simulink model "item3_simulink_motorCC_217947_222370"  (R2022a)
settings: Solver=VariableStepAuto  StartTime=0.0  StopTime=0.2  RelTol=1e-6
values from neighbouring files (symbols this model uses):
  Ia_placa = 25    [matlab_motorCC_217947_222370.m]
  J = 0.00252    [matlab_motorCC_217947_222370.m]
  K = Te_placa/Ia_placa    (= 0.424752712124)    [matlab_motorCC_217947_222370.m]
  Kac = 1/Kpc    (= 0.588235294118)    [matlab_motorCC_217947_222370.m]
  Kas = 1/Kps    (= 1.68552663541)    [matlab_motorCC_217947_222370.m]
  Kic = Ra*wcc    (= 260)    [matlab_motorCC_217947_222370.m]
  Kis = J*wcs^2/(5*K)    (= 11.8657276485)    [matlab_motorCC_217947_222370.m]
  Kpc = La*wcc    (= 1.7)    [matlab_motorCC_217947_222370.m]
  Kps = J*wcs/K    (= 0.593286382423)    [matlab_motorCC_217947_222370.m]
  La = 1.7e-3    (= 0.0017)    [matlab_motorCC_217947_222370.m]
  Ra = 0.26    [matlab_motorCC_217947_222370.m]
  Te_placa = Potencia/Wm_placa    (= 10.6188178031)    [matlab_motorCC_217947_222370.m]
  Va_placa = 140    [matlab_motorCC_217947_222370.m]
libraries: spsDCVoltageSourceLib x1, spsDCMachineLib x1, spsFullBridgeConverterLib x1, spsPWMGenerator2LevelLib x1, spspowerguiLib x1
settings Model: Creator=mathe  LastModifiedBy=Pichau

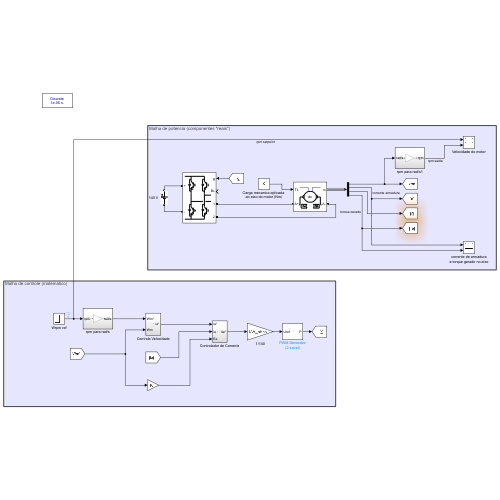
[thumbnail: Simulink's stored preview of the top-level diagram]
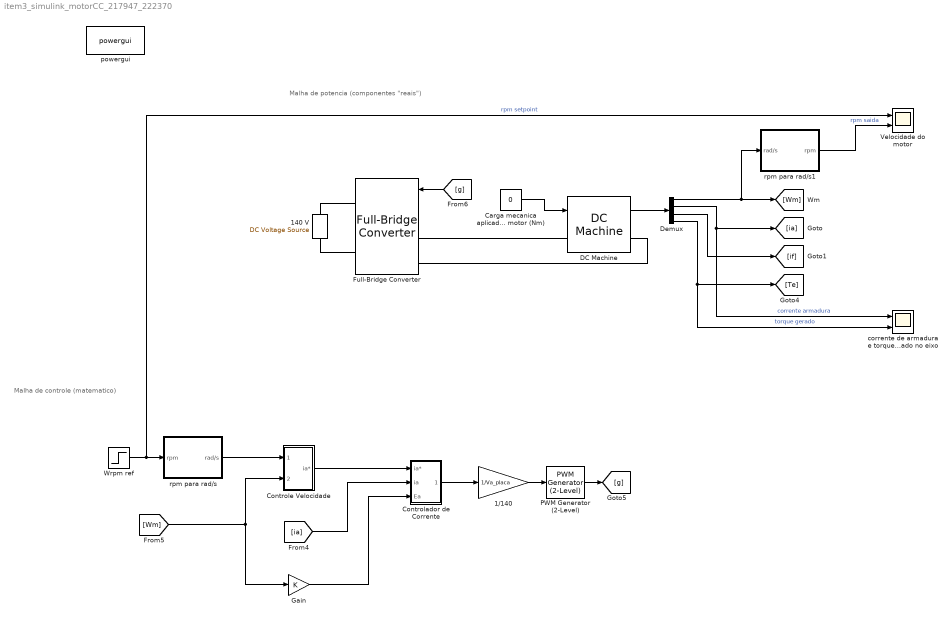
== system item3_simulink_motorCC_217947_222370 ==
  note: Malha de potencia (componentes "reais")
  note: Malha de controle (matematico)
  1/140 : Gain  Gain=1/Va_placa
  140 V : spsDCVoltageSourceLib/DC Voltage Source  Amplitude=Va_placa  Measurements=None
  Carga mecanica aplicada ao eixo do motor (Nm) : Constant  Value=0
  Controlador de Corrente : Subsystem
  Controle Velocidade : Subsystem
  DC Machine : spsDCMachineLib/DC Machine  PresetModel=No  MechanicalLoad=Torque TL  FieldType=Permanent magnet  ShowDetailedParameters=on  MeasurementBus=off  RLa="[ Ra  La]"  RLf="[ 240  120]"  Laf=1.8  MachineConstant=Torque constant (N.m/A)  Ke=1.8  Kt=K  J=J  Bm=B  Tf=0  w0=0  Ifinit=1  TsPowergui=0  TsBlock=-1
  Demux : Demux
  Full-Bridge Converter : spsFullBridgeConverterLib/Full-Bridge Converter  ModelType=Switching devices  Ron=1e-3  Rs=1e6  Cs=inf  Vforward=[0,0]  Ron_Diode=1e-3  Rs_Diode=1e6  Cs_Diode=inf  Vf_Diode=1e-3  Rs_CurrentSource=inf  Ron_ACsource=1e-3
      settings: SourceProductBaseCode=PS
  Gain : Gain  Gain=K
  PWM Generator (2-Level) : spsPWMGenerator2LevelLib/PWM Generator (2-Level)  ModulatorType=Single-phase full-bridge (4 pulses)  ModulatorMode=Unsynchronized  Fc=5000  Pc=90  nF=27  MinMax="[ 0  1 ]"  SamplingTechnique=Natural  ModulatingSignals=off  m=0.8  Freq=60  Phase=0  Ts=0  ShowCarrierOutport=off
  Velocidade do motor : Scope  NumInputPorts=2
  Wrpm ref : Step  Time=0.05  After=2500  SampleTime=0
  corrente de armadura e torque gerado no eixo : Scope  NumInputPorts=2
  powergui : spspowerguiLib/powergui  Priority=1  SimulationMode=Discrete  SampleTime=1e-6  frequency=60  Iterations=50  frequencyindice=0  Pbase=100e6  ErrMax=1e-4  UnitsV=kV  UnitsW=MW  buscounter=0  FunctionMessages=off  echomessages=off  EnableUseOfTLC=off  CurrentSourceSwitches=off  DisableSnubberDevices=off  DisableRonSwitches=off  DisableVfSwitches=off  DisplayEquations=off  AutomaticDiscreteSolvers=off  SolverType=Tustin/Backward Euler (TBE)  Interpol=off  ExternalGateDelay=off  methode=off  Ts=100  x0status=blocks  SPID=on  SwTol=0  HookPort=off  NonlinearTolerance=1e-4  nMaxIteration=100  ContinueOnMaxIteration=off  RestoreLinks=warning  ResistiveCurrentMeasurement=off  Frange=[0:2:500]  Ylog=off  Xlog=on  ShowGrid=off  save=off  variable=ZData  structure=0  ZoomFFT=off  StartTime=0.0  cycles=1  DisplayStyle=1  fundamental=60  FreqAxis=off  MaxFrequency=1000  frequencyindicesteady=1  RmsSteady=1  display=off
  rpm para rad/s : Subsystem
  rpm para rad/s1 : Subsystem
  wires:
  DC Machine/1 -> Demux/1
  Demux/1 -> rpm para rad/s1/1(rad/s), [Wm]
  Wrpm ref/1 -> rpm para rad/s/1(rpm), Velocidade do motor/1  "rpm setpoint"
  rpm para rad/s/1(rad/s) -> Controle Velocidade/1(Wm*)
  Controle Velocidade/1(ia*) -> Controlador de Corrente/1(ia*)
  [Wm] -> Gain/1, Controle Velocidade/2(Wm)
  Demux/2 -> corrente de armadura e torque gerado no eixo/1, [ia]  "corrente armadura"
  [ia] -> Controlador de Corrente/2(ia)
  Carga mecanica aplicada ao eixo do motor (Nm)/1 -> DC Machine/1
  Demux/3 -> [if]
  Gain/1 -> Controlador de Corrente/3(Ea)
  PWM Generator (2-Level)/1 -> [g]
  Demux/4 -> corrente de armadura e torque gerado no eixo/2, [Te]  "torque gerado"
  Controlador de Corrente/1(Va*) -> 1/140/1
  1/140/1 -> PWM Generator (2-Level)/1
  rpm para rad/s1/1(rpm) -> Velocidade do motor/2  "rpm saida"
  [g] -> Full-Bridge Converter/1
  connections:
  Full-Bridge Converter/LConn1 -- DC Machine/LConn1
  Full-Bridge Converter/LConn2 -- DC Machine/RConn1
  140 V/RConn1 -- Full-Bridge Converter/RConn1
  140 V/LConn1 -- Full-Bridge Converter/RConn2

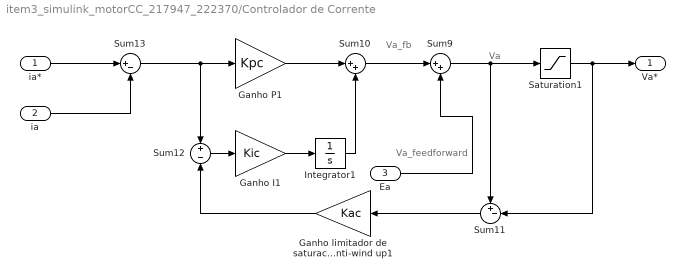
== system item3_simulink_motorCC_217947_222370/Controlador de Corrente ==
  note: Va
  note: Va_feedforward
  note: Va_fb
  ia* : Inport
  ia : Inport  Port=2
  Ea : Inport  Port=3
  Ganho I1 : Gain  Gain=Kic
  Ganho P1 : Gain  Gain=Kpc
  Ganho limitador de saturacao anti-wind up1 : Gain  Gain=Kac
  Integrator1 : Integrator
  Saturation1 : Saturate  UpperLimit=Va_placa  LowerLimit=-Va_placa
  Sum10 : Sum  Inputs=|++
  Sum11 : Sum  Inputs=+-|
  Sum12 : Sum  Inputs=+|-
  Sum13 : Sum  Inputs=|+-
  Sum9 : Sum  Inputs=|++
  Va* : Outport
  wires:
  Sum9/1 -> Sum11/1, Saturation1/1
  Sum10/1 -> Sum9/1
  Sum13/1 -> Sum12/1, Ganho P1/1
  Ganho P1/1 -> Sum10/1
  Sum12/1 -> Ganho I1/1
  Sum11/1 -> Ganho limitador de saturacao anti-wind up1/1
  Ganho I1/1 -> Integrator1/1
  ia*/1 -> Sum13/1
  Integrator1/1 -> Sum10/2
  Ganho limitador de saturacao anti-wind up1/1 -> Sum12/2
  Saturation1/1 -> Va*/1, Sum11/2
  ia/1 -> Sum13/2
  Ea/1 -> Sum9/2

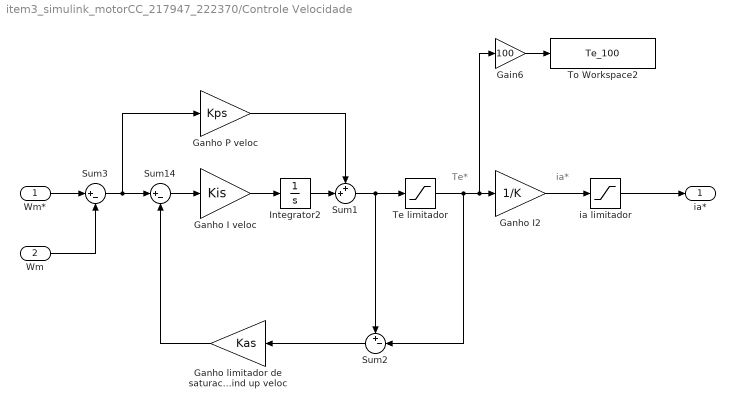
== system item3_simulink_motorCC_217947_222370/Controle Velocidade ==
  note: Te*
  note: ia*
  Wm* : Inport
  Wm : Inport  Port=2
  Gain6 : Gain  Gain=100
  Ganho I veloc : Gain  Gain=Kis
  Ganho I2 : Gain  Gain=1/K
  Ganho P veloc : Gain  Gain=Kps
  Ganho limitador de saturacao anti-wind up veloc : Gain  Gain=Kas
  Integrator2 : Integrator
  Sum1 : Sum  Inputs=++|
  Sum14 : Sum  Inputs=|+-
  Sum2 : Sum  Inputs=+-|
  Sum3 : Sum  Inputs=|+-
  Te limitador : Saturate  UpperLimit=Te_placa  LowerLimit=-Te_placa
  To Workspace2 : ToWorkspace  VariableName=Te_100  SaveFormat=Timeseries  SampleTime=-1
  ia limitador : Saturate  UpperLimit=Ia_placa  LowerLimit=-Ia_placa
  ia* : Outport
  wires:
  Ganho I2/1 -> ia limitador/1
  Sum3/1 -> Ganho P veloc/1, Sum14/1
  Sum14/1 -> Ganho I veloc/1
  Te limitador/1 -> Gain6/1, Ganho I2/1, Sum2/2
  Ganho limitador de saturacao anti-wind up veloc/1 -> Sum14/2
  Gain6/1 -> To Workspace2/1
  Ganho P veloc/1 -> Sum1/1
  Sum1/1 -> Sum2/1, Te limitador/1
  Integrator2/1 -> Sum1/2
  Wm*/1 -> Sum3/1
  Sum2/1 -> Ganho limitador de saturacao anti-wind up veloc/1
  Ganho I veloc/1 -> Integrator2/1
  ia limitador/1 -> ia*/1
  Wm/1 -> Sum3/2

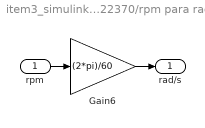
== system item3_simulink_motorCC_217947_222370/rpm para rad//s ==
  rpm : Inport
  Gain6 : Gain  Gain=(2*pi)/60
  rad/s : Outport
  wires:
  rpm/1 -> Gain6/1
  Gain6/1 -> rad/s/1

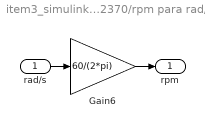
== system item3_simulink_motorCC_217947_222370/rpm para rad//s1 ==
  rad/s : Inport
  Gain6 : Gain  Gain=60/(2*pi)
  rpm : Outport
  wires:
  rad/s/1 -> Gain6/1
  Gain6/1 -> rpm/1
